simulink model "tarea3"  (R2015a)
settings: Solver=ode45  StartTime=0.0  StopTime=30  RelTol=1e-3
settings Model: Creator=Sala2  LastModifiedBy=Sala8

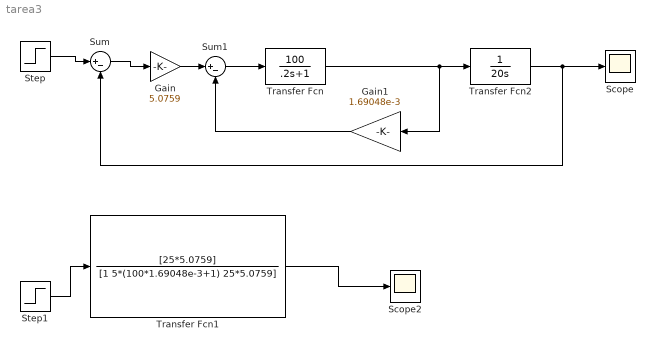
== system tarea3 ==
  Gain : Gain  Gain=5.0759
  Gain1 : Gain  Gain=1.69048e-3
  Scope : Scope
  Scope2 : Scope
      settings: SaveName=ScopeData2
  Step : Step  Time=0  SampleTime=0
  Step1 : Step  Time=0  SampleTime=0
  Sum : Sum  Inputs=|+-
  Sum1 : Sum  Inputs=|+-
  Transfer Fcn : TransferFcn  Numerator=[100]  Denominator=[.2 1]
  Transfer Fcn1 : TransferFcn  Numerator=[25*5.0759]  Denominator=[1 5*(100*1.69048e-3+1) 25*5.0759]
  Transfer Fcn2 : TransferFcn  Denominator=[20 0]
  wires:
  Step/1 -> Sum/1
  Sum/1 -> Gain/1
  Transfer Fcn/1 -> Gain1/1, Transfer Fcn2/1
  Gain/1 -> Sum1/1
  Sum1/1 -> Transfer Fcn/1
  Gain1/1 -> Sum1/2
  Transfer Fcn2/1 -> Sum/2, Scope/1
  Step1/1 -> Transfer Fcn1/1
  Transfer Fcn1/1 -> Scope2/1
